simulink model "scars_example2"  (R2019b)
settings: Solver=ode14x  StartTime=0.0  StopTime=20  FixedStep=dT  RelTol=1e-3
undefined symbols (not defined in the file or in its folder): Continuous, Time
libraries: scars_library x8, ctrlSharedLib x1, simulink x1
settings Model: Creator=asmialek  LastModifiedBy=asmialek

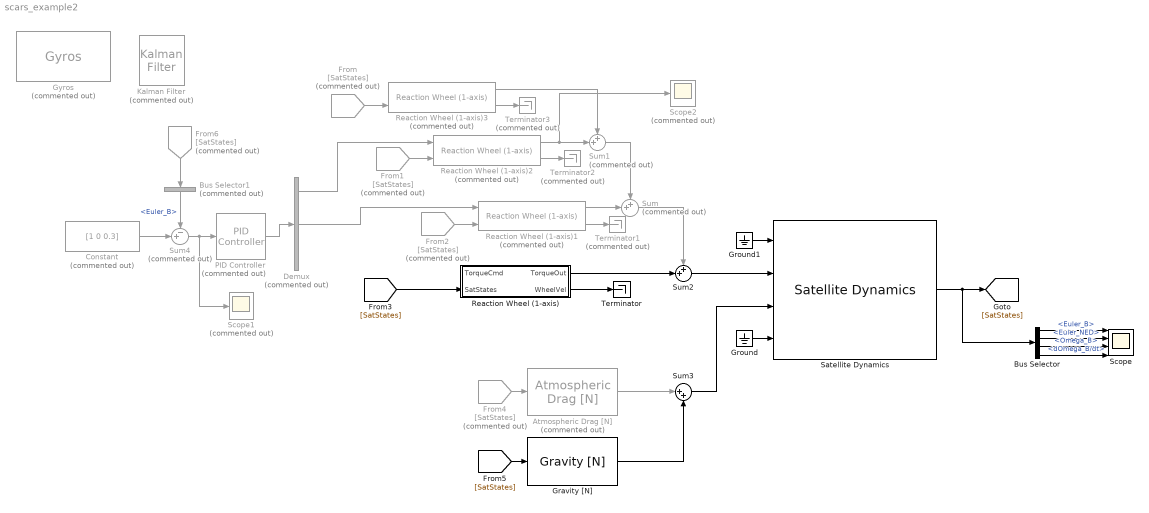
== system scars_example2 ==
  Atmospheric Drag [N] : scars_library/Environment/Atmospheric Drag [N]  Commented=on  SystemSampleTime=-1  Latency=0  AutoFrameSizeCalculation=off
  Bus Selector : BusSelector  OutputSignals=Euler_B,Euler_NED,Omega_B,dOmega_B/dt
  Bus Selector1 : BusSelector  Commented=on  OutputSignals=Euler_B
  Constant : Constant  Commented=on  Value=[1 0 0.3]
  Demux : Demux  Commented=on  Outputs=3
  From{,1..2,4,6} (5 alike) : From  Commented=on  GotoTag=SatStates
  Gravity [N] : scars_library/Environment/Gravity [N]  mass=5
  Ground : Ground
  Ground1 : Ground
  Gyros : scars_library/Sensors/Gyros  Commented=on  g_wn=1000*2*pi  g_w=12.5*2*pi  g_zeta=sqrt(2)/2  g_bias=0  g_z=1  g_max=0  g_min=0
  Kalman Filter : ctrlSharedLib/Kalman Filter  Commented=on  TimeDomain=Continuous-Time  UseCurrentEstimator=on  ModelSource=Individual A, B, C, D matrices  ModelSourceVariable=ss(0.95,1,1,0,1)  A=0.95  B=1  C=1  D=0  NumberOfStates=1  NumberOfInputs=1  NumberOfOutputs=1  InitialEstimateSource=Dialog  X0=0  P0=10  UseK=off  UseGH=off  NumberOfProcessNoiseInputs=1  G=1  TimeInvariantG=on  H=0  TimeInvariantH=on  Q=0.05  TimeInvariantQ=on  R=1  TimeInvariantR=on  N=0  TimeInvariantN=on  AddInputPort=on  AddEnablePort=off  OutputEstimatedY=off  OutputP=off  Ts=-1
      settings: SourceProductBaseCode=CT
  PID Controller : scars_library/ Control Algorithms /PID Controller  Commented=on  Kp=1  Ki=0.001  Kd=10  pid_sat_max=inf  pid_sat_min=-inf  pid_dz_max=0  pid_dz_min=0
  Reaction Wheel (1-axis) : Subsystem  AncestorBlock=scars_library/Actuators/Reaction Wheel (1-axis)  mask{axis_switch=Z, N=25e-3, R=0.1, J=1, c=0.0001, rw_power=0.0001, rw_freq=0.1}
      mask prompts: axis_switch "Operating Axis"; rw_power "Output Noise Power"; rw_freq "Noise Frequency"
      mask TypeOptions axis_switch: X | Y | Z
  Reaction Wheel (1-axis)1 : scars_library/Actuators/Reaction Wheel (1-axis)  Commented=on  axis_switch=Y  N=25e-3  R=0.1  J=1  c=0.0001  rw_power=0.0001  rw_freq=0.1  SSRTWFcnClass=[]
  Reaction Wheel (1-axis)2 : scars_library/Actuators/Reaction Wheel (1-axis)  Commented=on  axis_switch=X  N=25e-3  R=0.1  J=1  c=0.0001  rw_power=0.000001  rw_freq=0.1  SSRTWFcnClass=[]
  Reaction Wheel (1-axis)3 : scars_library/Actuators/Reaction Wheel (1-axis)  Commented=on  axis_switch=X  N=25e-3  R=0.1  J=1  c=0.0001  rw_power=0.0001  rw_freq=0.1  SSRTWFcnClass=[]
  Satellite Dynamics : scars_library/Advanced/Satellite Dynamics  Parameter4=Keplerian Elements  epoch=2451545  mass=5  a=6356e3+400e3  e=0  incl=30  RA=0  w=0  TA=30  initEuler=[47 12 63]  initEulerRates=[0.01 0.02 0.005]  TA_copy=0  TA_copy_copy=0
  Scope : Scope  NumInputPorts=4
  Scope1 : Scope  Commented=on
  Scope2 : Scope  Commented=on
  Sum : Sum  Commented=on  Inputs=++|
  Sum1 : Sum  Commented=on  Inputs=++|
  Sum2 : Sum  Inputs=++|
  Sum3 : Sum  Inputs=|++
  Sum4 : Sum  Commented=on  Inputs=-+|
  Terminator : Terminator
  Terminator1 : Terminator  Commented=on
  Terminator2 : Terminator  Commented=on
  Terminator3 : Terminator  Commented=on
  wires:
  Reaction Wheel (1-axis)/2(WheelVel) -> Terminator/1
  Reaction Wheel (1-axis)1/2 -> Terminator1/1
  Reaction Wheel (1-axis)2/2 -> Terminator2/1
  Reaction Wheel (1-axis)3/2 -> Terminator3/1
  Reaction Wheel (1-axis)1/1 -> Sum/2
  Reaction Wheel (1-axis)3/1 -> Sum1/1
  Sum1/1 -> Sum/1
  Sum/1 -> Sum2/1
  Satellite Dynamics/1 -> Bus Selector/1, [SatStates]
  From/1 -> Reaction Wheel (1-axis)3/2
  From1/1 -> Reaction Wheel (1-axis)2/2
  From2/1 -> Reaction Wheel (1-axis)1/2
  From4/1 -> Atmospheric Drag [N]/1
  [SatStates] -> Gravity [N]/1
  Atmospheric Drag [N]/1 -> Sum3/1
  Gravity [N]/1 -> Sum3/2
  Sum3/1 -> Satellite Dynamics/3
  Ground/1 -> Satellite Dynamics/4
  Ground1/1 -> Satellite Dynamics/1
  Bus Selector/1 -> Scope/1  "<Euler_B>"
  Bus Selector/2 -> Scope/2  "<Euler_NED>"
  Bus Selector/3 -> Scope/3  "<Omega_B>"
  Bus Selector/4 -> Scope/4  "<dOmega_B/dt>"
  Constant/1 -> Sum4/2
  Sum4/1 -> Scope1/1, PID Controller/1
  PID Controller/1 -> Demux/1
  Demux/1 -> Reaction Wheel (1-axis)2/1
  Demux/2 -> Reaction Wheel (1-axis)1/1
  From6/1 -> Bus Selector1/1
  Bus Selector1/1 -> Sum4/1  "<Euler_B>"
  Reaction Wheel (1-axis)2/1 -> Scope2/1, Sum1/2
  Sum2/1 -> Satellite Dynamics/2
  [SatStates] -> Reaction Wheel (1-axis)/2(SatStates)
  Reaction Wheel (1-axis)/1(TorqueOut) -> Sum2/2

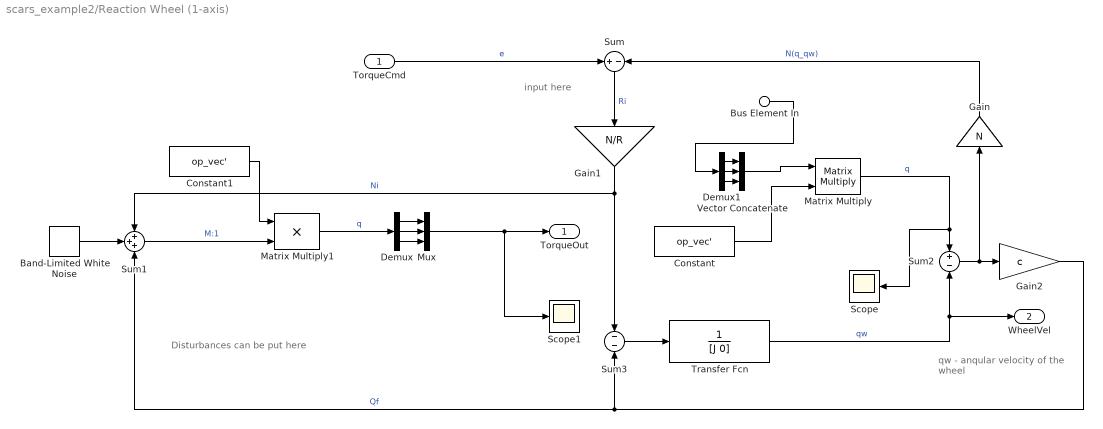
== system scars_example2/Reaction Wheel (1-axis) ==
  note: Disturbances can
      | be put here
  note: input here
  note: qw - anqular velocity
      |  of the wheel
  TorqueCmd : Inport
  Bus Element In : Inport  Port=2  PortName=SatStates  Element=Omega_B
  Band-Limited White Noise : simulink/Sources/Band-Limited White Noise  Cov=rw_power  Ts=rw_freq  seed=[23341]
  Constant : Constant  Value=op_vec'  VectorParams1D=off
  Constant1 : Constant  Value=op_vec'  VectorParams1D=off
  Demux : Demux  Outputs=3
  Demux1 : Demux  Outputs=3
  Gain : Gain  Gain=N
  Gain1 : Gain  Gain=N/R
  Gain2 : Gain  Gain=c
  Matrix Multiply : Product  Multiplication=Matrix(*)
  Matrix Multiply1 : Product
  Mux : Mux  Inputs=3
  Scope : Scope
  Scope1 : Scope
  Sum : Sum  Inputs=+|-
  Sum1 : Sum  Inputs=+++
  Sum2 : Sum  Inputs=+|-
  Sum3 : Sum  Inputs=-|-
  Transfer Fcn : TransferFcn  Denominator=[J 0]
  Vector Concatenate : Concatenate  NumInputs=3
  TorqueOut : Outport
  WheelVel : Outport  Port=2
  wires:
  Band-Limited White Noise/1 -> Sum1/2
  Gain1/1 -> Sum1/1, Sum3/1  "Ni"
  TorqueCmd/1 -> Sum/1  "e"
  Sum3/1 -> Transfer Fcn/1
  Sum/1 -> Gain1/1  "Ri"
  Transfer Fcn/1 -> Sum2/2, WheelVel/1  "qw"
  Gain2/1 -> Sum3/2, Sum1/3  "Qf"
  Sum1/1 -> Matrix Multiply1/2  "M:1"
  Sum2/1 -> Gain2/1, Gain/1
  Gain/1 -> Sum/2  "N(q_qw)"
  Matrix Multiply/1 -> Scope/1, Sum2/1  "q"
  Constant1/1 -> Matrix Multiply1/1
  Constant/1 -> Matrix Multiply/2
  Matrix Multiply1/1 -> Demux/1  "q"
  Mux/1 -> Scope1/1, TorqueOut/1
  Demux/1 -> Mux/1
  Demux/2 -> Mux/2
  Demux/3 -> Mux/3
  Demux1/1 -> Vector Concatenate/1
  Demux1/2 -> Vector Concatenate/2
  Demux1/3 -> Vector Concatenate/3
  Bus Element In/1 -> Demux1/1
  Vector Concatenate/1 -> Matrix Multiply/1
